simulink model "model3"  (R2014a)
settings: Solver=ode45  StartTime=0.0  StopTime=10.0  RelTol=1e-3
libraries: simulink x1
settings Model: Creator=Javier  LastModifiedBy=Javier

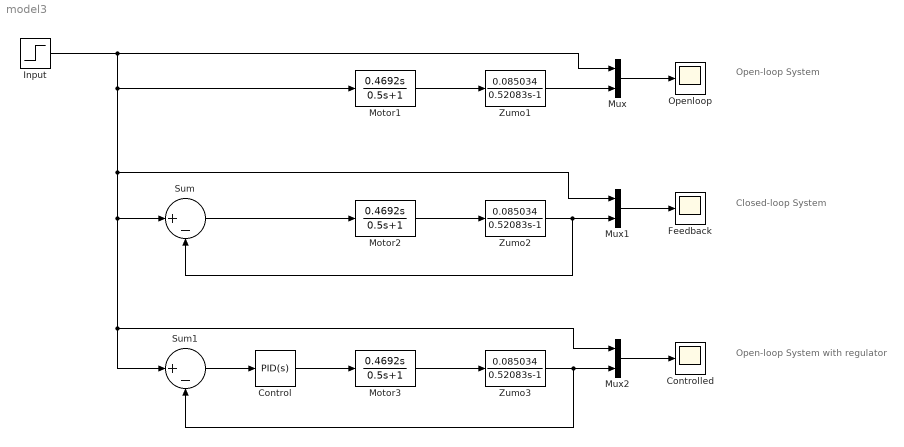
== system model3 ==
  note: Open-loop System
  note: Closed-loop System
  note: Open-loop System with regulator
  Control : simulink/Continuous/PID Controller  Controller=PID  TimeDomain=Continuous-time  SampleTime=1  IntegratorMethod=Forward Euler  FilterMethod=Forward Euler  Form=Parallel  P=1  I=1  D=0  N=100  InitialConditionSource=internal  InitialConditionForIntegrator=0  InitialConditionForFilter=0  ExternalReset=none  LimitOutput=off  UpperSaturationLimit=inf  LowerSaturationLimit=-inf  LinearizeAsGain=on  AntiWindupMode=none  Kb=1  TrackingMode=off  Kt=1  PParamMin=[]  PParamMax=[]  IParamMin=[]  IParamMax=[]  DParamMin=[]  DParamMax=[]  NParamMin=[]  NParamMax=[]  KbParamMin=[]  KbParamMax=[]  KtParamMin=[]  KtParamMax=[]  POutMin=[]  POutMax=[]  IOutMin=[]  IOutMax=[]  DOutMin=[]  DOutMax=[]  NOutMin=[]  NOutMax=[]  KbOutMin=[]  KbOutMax=[]  KtOutMin=[]  KtOutMax=[]  IntegratorOutMin=[]  IntegratorOutMax=[]  FilterOutMin=[]  FilterOutMax=[]  SumOutMin=[]  SumOutMax=[]  SumI1OutMin=[]  SumI1OutMax=[]  SumI2OutMin=[]  SumI2OutMax=[]  SumI3OutMin=[]  SumI3OutMax=[]  SumDOutMin=[]  SumDOutMax=[]  SaturationOutMin=[]  SaturationOutMax=[]  IntegratorContinuousStateAttributes=''  IntegratorStateMustResolveToSignalObject=off  IntegratorRTWStateStorageClass=Auto  FilterContinuousStateAttributes=''  FilterStateMustResolveToSignalObject=off  FilterRTWStateStorageClass=Auto
  Controlled : Scope
      settings: SaveName=ScopeData2
  Feedback : Scope
  Input : Step  SampleTime=0
  Motor1 : TransferFcn  Numerator=[0.4692 0]  Denominator=[0.5 1]
  Motor2 : TransferFcn  Numerator=[0.4692 0]  Denominator=[0.5 1]
  Motor3 : TransferFcn  Numerator=[0.4692 0]  Denominator=[0.5 1]
  Mux : Mux  Inputs=2
  Mux1 : Mux  Inputs=2
  Mux2 : Mux  Inputs=2
  Openloop : Scope
  Sum : Sum  Inputs=|+-
  Sum1 : Sum  Inputs=|+-
  Zumo1 : TransferFcn  Numerator=[0.085034]  Denominator=[0.52083 -1]
  Zumo2 : TransferFcn  Numerator=[0.085034]  Denominator=[0.52083 -1]
  Zumo3 : TransferFcn  Numerator=[0.085034]  Denominator=[0.52083 -1]
  wires:
  Zumo1/1 -> Mux/2
  Motor1/1 -> Zumo1/1
  Input/1 -> Mux/1, Motor1/1, Mux1/1, Sum1/1, Mux2/1, Sum/1
  Sum/1 -> Motor2/1
  Motor2/1 -> Zumo2/1
  Zumo2/1 -> Mux1/2, Sum/2
  Mux1/1 -> Feedback/1
  Mux/1 -> Openloop/1
  Motor3/1 -> Zumo3/1
  Control/1 -> Motor3/1
  Sum1/1 -> Control/1
  Zumo3/1 -> Sum1/2, Mux2/2
  Mux2/1 -> Controlled/1
